simulink model "Optimal_Simulation_ICE"  (R2020a)
settings: Solver=ode45  StartTime=0.0  StopTime=6948  RelTol=1e-3
values from neighbouring files (symbols this model uses):
  diff_gear = x(7)    [Opti_sub_ICE.m]
  do_21 = x(13)    [Opti_sub_ICE.m]
  do_32 = x(14)    [Opti_sub_ICE.m]
  do_43 = x(15)    [Opti_sub_ICE.m]
  do_54 = x(16)    [Opti_sub_ICE.m]
  do_65 = x(17)    [Opti_sub_ICE.m]
  EM_gear_ratio = 4.51    [init_Opti_ICE.m]
  fifth_gear = x(5)    [Opti_sub_ICE.m]
  first_gear = x(1)    [Opti_sub_ICE.m]
  fourth_gear = x(4)    [Opti_sub_ICE.m]
  gear_eff = 0.95    [init_Opti_ICE.m]
  gear_idling_loss = 300    [init_Opti_ICE.m]
  max_CE_power = 60    [init_Opti_ICE.m]
  max_EM_power = 90    [init_Opti_ICE.m]
  max_SOC = 0.60    (= 0.6)    [init_Opti_ICE.m]
  min_SOC = 0.35    [init_Opti_ICE.m]
  second_gear = x(2)    [Opti_sub_ICE.m]
  sixth_gear = x(6)    [Opti_sub_ICE.m]
  T_CE_max = p_me_max*V_d/(2*pi*2)    [init_Opti_ICE.m]
  T_EM_max = T_EM_max * max_EM_power*1000/max_EM_power_old    [init_Opti_ICE.m]
  third_gear = x(3)    [Opti_sub_ICE.m]
  up_12 = x(8)    [Opti_sub_ICE.m]
  up_23 = x(9)    [Opti_sub_ICE.m]
  up_34 = x(10)    [Opti_sub_ICE.m]
  up_45 = x(11)    [Opti_sub_ICE.m]
  up_56 = x(12)    [Opti_sub_ICE.m]
  V_wheel_dia = 0.739    [init_Opti_ICE.m]
undefined symbols (not defined in the file or in its folder): automatic_gearbox, eta_EM_map, h, H_u, k_cs, P_aux, P_CE_cutoff, P_CE_idle, r, rho_f, T_CE_cutoff, theta_CE, theta_EM, V_CE_map, w_CE_idle, w_CE_max, w_CE_upper, w_EM_row, w_EM_upper
libraries: qss_tb_library x5
settings Model: Creator=davidci  LastModifiedBy=Rahul Pai
settings DataIOCC: LimitDataPoints=on  SaveFormat=Array  ReturnWorkspaceOutputs=off
settings OptimizationCC: BlockReduction=off  BooleanDataType=off  LifeSpan=inf
settings DebuggingCC: SaveWithParameterizedLinksMsg=none  UnderspecifiedInitializationDetection=Classic  MergeDetectMultiDrivingBlocksExec=none  SignalResolutionControl=TryResolveAllWithWarning  SFUnexpectedBacktrackingDiag=warning  SFNoUnconditionalDefaultTransitionDiag=warning  SFExecutionAtInitializationDiag=none  ArithmeticOperatorsInVariantConditions=warning
settings HardwareCC: ProdBitPerPointer=32  ProdBitPerSizeT=32  ProdBitPerPtrDiffT=32  ProdLargestAtomicFloat=None  ProdIntDivRoundTo=Undefined  ProdEndianess=Unspecified  ProdWordSize=32  ProdHWDeviceType=32-bit Generic  TargetUnknown=on
settings ModelReferenceCC: PropagateSignalLabelsOutOfModel=off
settings SFSimCC: SimUseLocalCustomCode=off  CustomCodeUndefinedFunction=UseInterfaceOnly
settings RTWCC: RTWUseLocalCustomCode=off
settings CodeAppCC: StateflowObjectComments=on
settings GRTTargetCC: TargetLangStandard=C89/C90 (ANSI)
settings ConfigComp: CovMetricSettings=dw  CovHtmlReporting=on  CovSaveCumulativeToWorkspaceVar=on  CovSaveSingleToWorkspaceVar=on  CovExternalEMLEnable=off  CovSFcnEnable=off

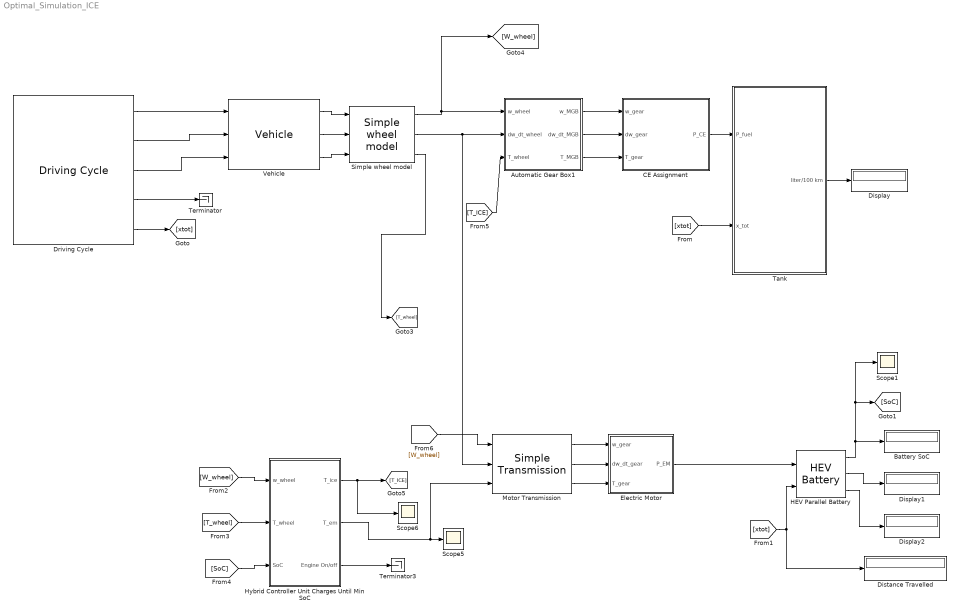
== system Optimal_Simulation_ICE ==
  Automatic Gear Box1 : Subsystem  Tag=transmission  AncestorBlock=qss_tb_library/Gear System/Automatic Gear Box  mask(Automatic Gear Box){nog=6, i=[first_gear second_gear third_gear fourth_gear fifth_gear sixth_gear], i_diff=diff_gear, gearon=[up_12 up_23 up_34 up_45 up_56], gearoff=[do_21 do_32 do_43 do_54 do_65], d=V_wheel_dia, e_GT=gear_eff, P_GT0=gear_idling_loss, w_wheel_min=1}
      mask prompts: nog "Number of gears"; i "Gear ratio vector"; i_diff "Differential gear [-]"; gearon "Switching points for upshift [km/h]"; gearoff "Switching points for downshift [km/h]"; d "Wheel diameter"; e_GT "Efficiency [-]"; P_GT0 "Idling losses (friction) [W]"; w_wheel_min "Minimum wheel speed beyond which losses are generated [rad/s]"
      mask help:
      | This block simulates a automatic gear box, can handle up to 16 gears.
      |
      | Input:
      | =====
      | 	w_wheel	Speed of the wheel [rad/s]
      | 	dw_dt_wheel	Acceleration of the wheel [rad/s^2],
      | 	T_wheel	Torque on the wheel [Nm]
      | 	i	Gear number [-]
      |
      | Output:
      | ======
      | 	w_MGB	Speed of the fly wheel [rad/s]
      | 	dw_dt_MGB	Acceleration of the fly wheel [rad/s^2]
      | 	T_MGB	Torque on the fly wheel [Nm]
      |
      | Number of gears:
      | ======
      | Specify the number of forward gears
      |
      | Shifting points for upshift:
      | ======
      | Vector specifying the velocity for shifting
      | [first_to_second_gear    second_to_third_gear    ....]
      | The number of elements in the vector should be Number of gears - 1.
      |
      | Shifting points for udownshift:
      | ======
      | Simular to upshift
      | [second_to_first_gear    third_to_second_gear    ....]
      mask init:
      | init_AGB;
  Battery SoC : Display
  CE Assignment : Subsystem  Tag=combustion engine  AncestorBlock=qss_tb_library/Energy Converter/CE Assignment  mask(Combustion Engine (based on consumption map)){engine_type=Gasoline, P_ice=max_CE_power, ENABLE_FUEL_CUTOFF=off}
      mask prompts: engine_type "Engine type"; P_ice "Power [kW]"; ENABLE_FUEL_CUTOFF "Enable fuel cutoff"
      mask help:
      | This block simulates the behaviour of a combustion engine. The block is based on consumption maps for medium sized passenger cars.
      |
      | NA Gasoline:
      | max power @ 5000 rpm
      | max torque @ 3000 rpm
      |
      | Small Diesel:
      | max power @ 4500 rpm
      | max torque @ 2000 rpm
      |
      | Large Diesel:
      | max power @ 1500 rpm
      | max torque @ 1500 rpm
      |
      |
      | Input:
      | =====
      | 	w_gear		Speed of the fly wheel [rad/s]
      | 	dw_gear	Acceleration of the fly wheel [rad/s^2]
      | 	T_gear		Torque on the fly wheel [Nm]
      |
      | Output:
      | ======
      | 	P_CE		Power produced by the combustion engine [W]
      mask init:
      | init_AssCE_map;
      mask TypeOptions engine_type: Gasoline | Small Diesel | Large Diesel
  Display : Display
  Display1 : Display
  Display2 : Display
  Distance Travelled : Display
      settings: Format=decimal (Stored Integer)
  Driving Cycle : qss_tb_library/Driving Cycle/Driving Cycle  Tag=cycle  cyclename1=Assignment_2_cycle  stepsize=1  autostop=on
  Electric Motor : Subsystem  AncestorBlock=qss_tb_library/Energy Converter/EM Assignment  mask(Electric Motor){P_em=max_EM_power}
      mask prompts: P_em "Power [kW]"
      mask help:
      | This block simulates the behaviour of an electric motor. The block is based on an efficiency map. The map is located in the Data/EnergyConvertter/ElectricMotor directory.
      |
      | Maximum speed och the electric motor is 6000 rpm
      | Field weakening region starts at 1500 rpm
      | Maximum mechanical power is at 2150 rpm
      | The maximum torque is 5.98 Nm/kW multiplied with the power you select.
      |
      | Input:
      | =====
      | 	w_gear	Speed of the motor [rad/s]
      | 	dw_dt_gear	Acceleration of the motor [rad/s^2]
      | 	T_gear	Torque of the motor [Nm]
      |
      | Output:
      | ======
      | 	P_EM	Electric Power consumed by the  motor [W]
      mask init:
      | init_EM_ass;
  HEV Parallel Battery : qss_tb_library/Energy Buffer/HEV Battery  Tag=battery  cell_series=N_series  cell_parallel=N_parallel  Q_BT_IC_rel=Init_SoC
  Hybrid Controller Unit Charges Until Min SoC : Subsystem  AncestorBlock=|  mask(Hybrid Controller Unit){}
      | qss_tb_library/Controller/Hybrid Controller Unit 
      | (Parallel, empty)
      mask help: Design your control strategy in this block.
      mask init:
      | init_HCU_parallel;
  Motor Transmission : qss_tb_library/Gear System/Simple Transmission  Tag=simple transmission  gear_ratio=EM_gear_ratio  e_GT=EM_gear_eta  P_GT0=EM_idling_loss  w_wheel_min=1
  Scope1 : Scope
  Scope5 : Scope
  Scope6 : Scope
  Simple wheel model : qss_tb_library/Vehicle/Simple wheel model  Tag=simple transmission  d_wheel=V_wheel_dia
  Tank : Subsystem  Tag=tank  AncestorBlock=qss_tb_library/Energy Source/Tank  mask(Tank){fuel=Gasoline, flag_cold_start=on}
      mask prompts: flag_cold_start "Include cold start losses"
      mask help:
      | This block integrates the power (the fuel mass flow) required by the combustion engine or the fuel cell and calculates the energy consumption in liter/100 km.
      |
      | Input:
      | =====
      | 	P_fuel	Power (fuel mass flow) required [W]
      | 	x_tot	Total distance [m]
      |
      | Output:
      | ======
      | 	V	Fuel consumption [liter/100 km]
      mask init:
      | init_tank;
      mask TypeOptions fuel: Gasoline | Diesel | Hydrogen
  Terminator : Terminator
  Terminator3 : Terminator
  Vehicle : qss_tb_library/Vehicle/Vehicle  Tag=vehicle  m_f=V_Mass  A_f=V_area  cw=V_d  mu=V_RRC  k_inertia=V_Rotating
  wires:
  Tank/1(liter/100 km) -> Display/1
  Driving Cycle/1 -> Vehicle/1
  Driving Cycle/2 -> Vehicle/2
  CE Assignment/1(P_CE) -> Tank/1(P_fuel)
  Driving Cycle/4 -> Terminator/1
  Driving Cycle/3 -> Vehicle/3
  Vehicle/1 -> Simple wheel model/1
  Vehicle/2 -> Simple wheel model/2
  Vehicle/3 -> Simple wheel model/3
  Automatic Gear Box1/3(T_MGB) -> CE Assignment/3(T_gear)
  Automatic Gear Box1/2(dw_dt_MGB) -> CE Assignment/2(dw_gear)
  Automatic Gear Box1/1(w_MGB) -> CE Assignment/1(w_gear)
  Simple wheel model/1 -> Automatic Gear Box1/1(w_wheel), [W_wheel]
  Simple wheel model/3 -> [T_wheel]
  Driving Cycle/5 -> [xtot]
  HEV Parallel Battery/3 -> Display2/1
  Motor Transmission/3 -> Electric Motor/3(T_gear)
  Motor Transmission/1 -> Electric Motor/1(w_gear)
  Hybrid Controller Unit Charges Until Min SoC/3(Engine On/off) -> Terminator3/1
  Motor Transmission/2 -> Electric Motor/2(dw_dt_gear)
  [xtot] -> HEV Parallel Battery/2, Distance Travelled/1
  Hybrid Controller Unit Charges Until Min SoC/2(T_em) -> Motor Transmission/3, Scope5/1
  Hybrid Controller Unit Charges Until Min SoC/1(T_ice) -> Scope6/1, [T_ICE]
  [SoC] -> Hybrid Controller Unit Charges Until Min SoC/3(SoC)
  Simple wheel model/2 -> Automatic Gear Box1/2(dw_dt_wheel), Motor Transmission/2
  HEV Parallel Battery/1 -> Scope1/1, [SoC], Battery SoC/1
  Electric Motor/1(P_EM) -> HEV Parallel Battery/1
  [W_wheel] -> Hybrid Controller Unit Charges Until Min SoC/1(w_wheel)
  [W_wheel] -> Motor Transmission/1
  [T_wheel] -> Hybrid Controller Unit Charges Until Min SoC/2(T_wheel)
  HEV Parallel Battery/2 -> Display1/1
  [T_ICE] -> Automatic Gear Box1/3(T_wheel)
  [xtot] -> Tank/2(x_tot)

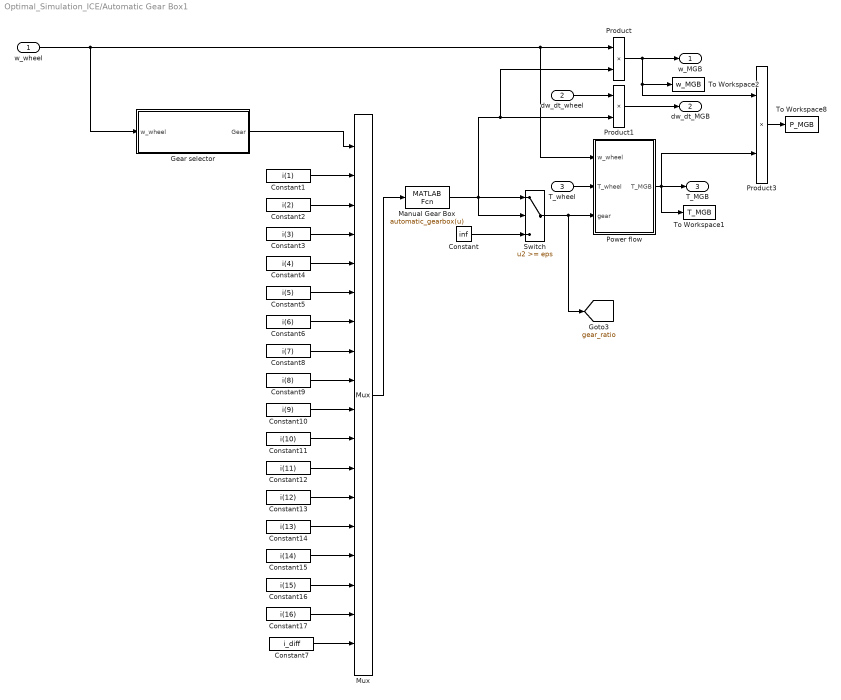
== system Optimal_Simulation_ICE/Automatic Gear Box1 ==
  w_wheel : Inport
  dw_dt_wheel : Inport  Port=2
  T_wheel : Inport  Port=3
  Constant : Constant  Value=inf
  Constant1 : Constant  Value=i(1)
  Constant10 : Constant  Value=i(9)
  Constant11 : Constant  Value=i(10)
  Constant12 : Constant  Value=i(11)
  Constant13 : Constant  Value=i(12)
  Constant14 : Constant  Value=i(13)
  Constant15 : Constant  Value=i(14)
  Constant16 : Constant  Value=i(15)
  Constant17 : Constant  Value=i(16)
  Constant2 : Constant  Value=i(2)
  Constant3 : Constant  Value=i(3)
  Constant4 : Constant  Value=i(4)
  Constant5 : Constant  Value=i(5)
  Constant6 : Constant  Value=i(6)
  Constant7 : Constant  Value=i_diff
  Constant8 : Constant  Value=i(7)
  Constant9 : Constant  Value=i(8)
  Gear selector : Subsystem
  Manual Gear Box : MATLABFcn  MATLABFcn=automatic_gearbox(u)  OutputDimensions=1
  Mux : Mux  Inputs=18
  Power flow : Subsystem
  Product : Product  InputSameDT=on  RndMeth=Zero  SaturateOnIntegerOverflow=on  OutDataTypeStr=Inherit: Same as first input
  Product1 : Product  InputSameDT=on  RndMeth=Zero  SaturateOnIntegerOverflow=on  OutDataTypeStr=Inherit: Same as first input
  Product3 : Product  InputSameDT=on  RndMeth=Zero  SaturateOnIntegerOverflow=on  OutDataTypeStr=Inherit: Same as first input
  Switch : Switch  Threshold=eps  SaturateOnIntegerOverflow=on  InputSameDT=on
  To Workspace1 : ToWorkspace  VariableName=T_MGB  SampleTime=-1
  To Workspace2 : ToWorkspace  VariableName=w_MGB  SampleTime=-1
  To Workspace8 : ToWorkspace  VariableName=P_MGB  SampleTime=-1
  w_MGB : Outport  InitialOutput=0
  dw_dt_MGB : Outport  Port=2  InitialOutput=0
  T_MGB : Outport  Port=3  InitialOutput=0
  tag scope: gear_ratio=global
  wires:
  Constant17/1 -> Mux/17
  Constant16/1 -> Mux/16
  Constant15/1 -> Mux/15
  Constant14/1 -> Mux/14
  Constant13/1 -> Mux/13
  Constant12/1 -> Mux/12
  Constant11/1 -> Mux/11
  Constant10/1 -> Mux/10
  Constant9/1 -> Mux/9
  Constant8/1 -> Mux/8
  Constant7/1 -> Mux/18
  Power flow/1(T_MGB) -> T_MGB/1, Product3/2, To Workspace1/1
  Product/1 -> w_MGB/1, Product3/1, To Workspace2/1
  Constant/1 -> Switch/3
  w_wheel/1 -> Gear selector/1(w_wheel), Product/1, Power flow/1(w_wheel)
  Product1/1 -> dw_dt_MGB/1
  dw_dt_wheel/1 -> Product1/1
  Manual Gear Box/1 -> Product/2, Product1/2, Switch/2, Switch/1
  Product3/1 -> To Workspace8/1
  Switch/1 -> [gear_ratio], Power flow/3(gear)
  T_wheel/1 -> Power flow/2(T_wheel)
  Constant1/1 -> Mux/2
  Constant2/1 -> Mux/3
  Constant3/1 -> Mux/4
  Constant4/1 -> Mux/5
  Constant5/1 -> Mux/6
  Constant6/1 -> Mux/7
  Gear selector/1(Gear) -> Mux/1
  Mux/1 -> Manual Gear Box/1

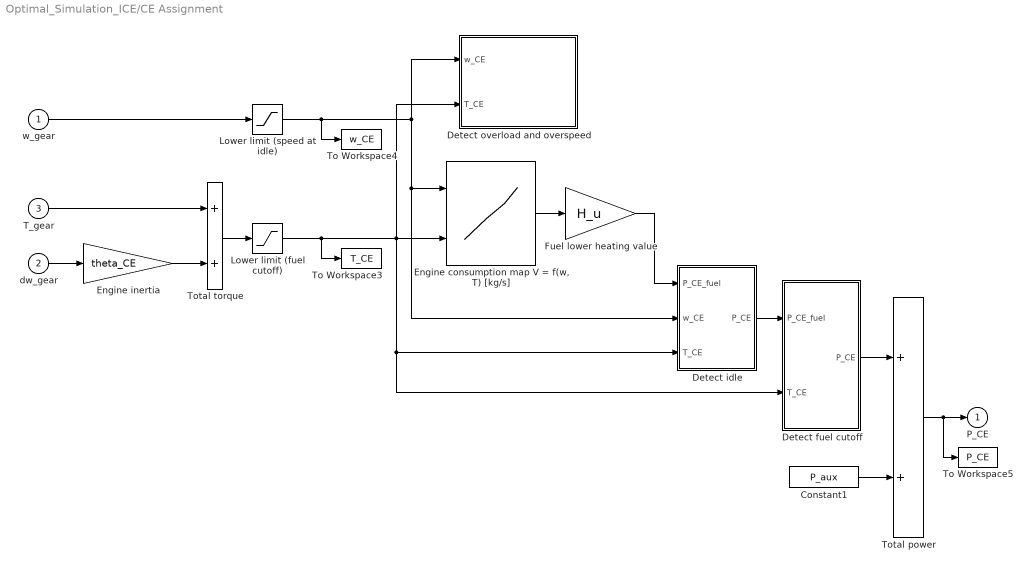
== system Optimal_Simulation_ICE/CE Assignment ==
  w_gear : Inport
  dw_gear : Inport  Port=2
  T_gear : Inport  Port=3
  Constant1 : Constant  Value=P_aux
  Detect fuel cutoff : Subsystem
  Detect idle : Subsystem
  Detect overload and overspeed : Subsystem
  "Engine consumption map V = f(w, T) [kg/s]" : Lookup2D  RowIndex=w_CE_row  ColumnIndex=T_CE_col  Table=V_CE_map
  Engine inertia : Gain  Gain=theta_CE  SaturateOnIntegerOverflow=on  OutDataTypeStr=Inherit: Same as input  ParamDataTypeStr=Inherit: Same as input
  Fuel lower heating value : Gain  Gain=H_u  SaturateOnIntegerOverflow=on  OutDataTypeStr=Inherit: Same as input  ParamDataTypeStr=Inherit: Same as input
  Lower limit (fuel cutoff) : Saturate  UpperLimit=inf  LowerLimit=T_CE_cutoff
  Lower limit (speed at idle) : Saturate  UpperLimit=inf  LowerLimit=w_CE_idle
  To Workspace3 : ToWorkspace  VariableName=T_CE  SampleTime=-1
  To Workspace4 : ToWorkspace  VariableName=w_CE  SampleTime=-1
  To Workspace5 : ToWorkspace  VariableName=P_CE  SampleTime=-1
  Total power : Sum  InputSameDT=on  SaturateOnIntegerOverflow=on  OutDataTypeStr=Inherit: Same as first input
  Total torque : Sum  InputSameDT=on  SaturateOnIntegerOverflow=on  OutDataTypeStr=Inherit: Same as first input
  P_CE : Outport  InitialOutput=0
  wires:
  T_gear/1 -> Total torque/1
  dw_gear/1 -> Engine inertia/1
  Total torque/1 -> Lower limit (fuel cutoff)/1
  Engine inertia/1 -> Total torque/2
  Lower limit (speed at idle)/1 -> Detect overload and overspeed/1(w_CE), Detect idle/2(w_CE), "Engine consumption map V = f(w, T) [kg/s]"/1, To Workspace4/1
  w_gear/1 -> Lower limit (speed at idle)/1
  Fuel lower heating value/1 -> Detect idle/1(P_CE_fuel)
  Detect idle/1(P_CE) -> Detect fuel cutoff/1(P_CE_fuel)
  "Engine consumption map V = f(w, T) [kg/s]"/1 -> Fuel lower heating value/1
  Detect fuel cutoff/1(P_CE) -> Total power/1
  Total power/1 -> P_CE/1, To Workspace5/1
  Constant1/1 -> Total power/2
  Lower limit (fuel cutoff)/1 -> Detect overload and overspeed/2(T_CE), "Engine consumption map V = f(w, T) [kg/s]"/2, Detect idle/3(T_CE), Detect fuel cutoff/2(T_CE), To Workspace3/1

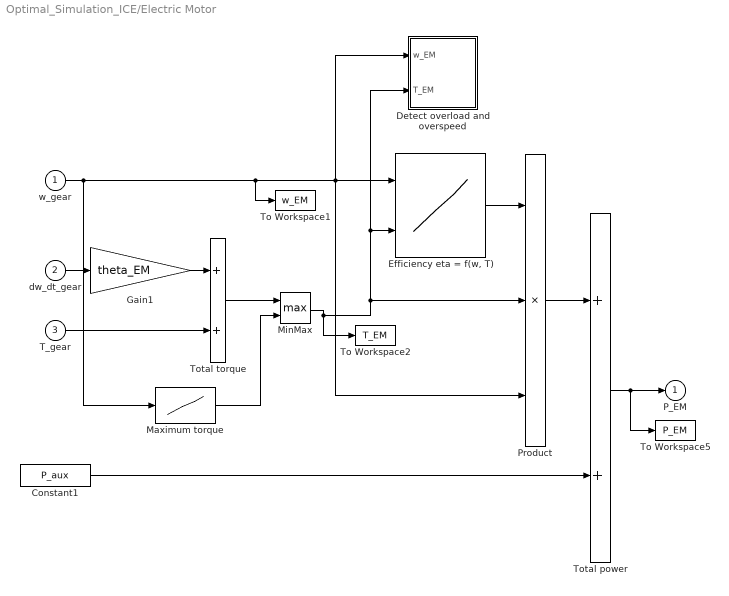
== system Optimal_Simulation_ICE/Electric Motor ==
  w_gear : Inport
  dw_dt_gear : Inport  Port=2
  T_gear : Inport  Port=3
  Constant1 : Constant  Value=P_aux
  Detect overload and overspeed : Subsystem
  "Efficiency eta = f(w, T)" : Lookup2D  RowIndex=w_EM_row  ColumnIndex=T_EM_col  Table=eta_EM_map
  Gain1 : Gain  Gain=theta_EM  SaturateOnIntegerOverflow=on  OutDataTypeStr=Inherit: Same as input  ParamDataTypeStr=Inherit: Same as input
  Maximum torque : Lookup  InputValues=w_EM_row  Table=-T_EM_max  SaturateOnIntegerOverflow=on
  MinMax : MinMax  Function=max  Inputs=2
  Product : Product  Inputs=3  InputSameDT=on  RndMeth=Zero  SaturateOnIntegerOverflow=on  OutDataTypeStr=Inherit: Same as first input
  To Workspace1 : ToWorkspace  VariableName=w_EM  SampleTime=-1
  To Workspace2 : ToWorkspace  VariableName=T_EM  SampleTime=-1
  To Workspace5 : ToWorkspace  VariableName=P_EM  SampleTime=-1
  Total power : Sum  InputSameDT=on  SaturateOnIntegerOverflow=on  OutDataTypeStr=Inherit: Same as first input
  Total torque : Sum  InputSameDT=on  SaturateOnIntegerOverflow=on  OutDataTypeStr=Inherit: Same as first input
  P_EM : Outport  InitialOutput=0
  wires:
  Total power/1 -> To Workspace5/1, P_EM/1
  Product/1 -> Total power/1
  Constant1/1 -> Total power/2
  MinMax/1 -> To Workspace2/1, Product/2, "Efficiency eta = f(w, T)"/2, Detect overload and overspeed/2(T_EM)
  Gain1/1 -> Total torque/1
  T_gear/1 -> Total torque/2
  dw_dt_gear/1 -> Gain1/1
  "Efficiency eta = f(w, T)"/1 -> Product/1
  w_gear/1 -> Maximum torque/1, To Workspace1/1, Product/3, "Efficiency eta = f(w, T)"/1, Detect overload and overspeed/1(w_EM)
  Maximum torque/1 -> MinMax/2
  Total torque/1 -> MinMax/1

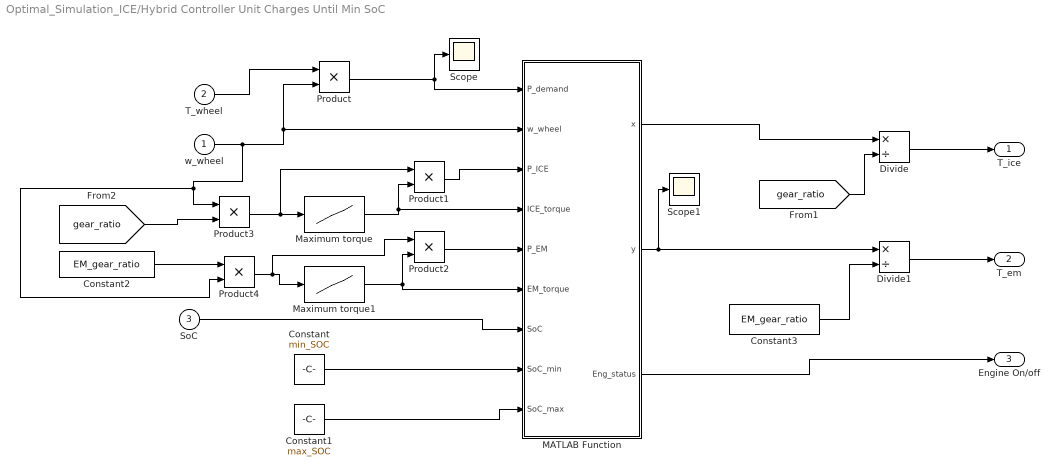
== system Optimal_Simulation_ICE/Hybrid Controller Unit Charges Until Min SoC ==
  w_wheel : Inport
  T_wheel : Inport  Port=2
  SoC : Inport  Port=3
  Constant : Constant  Value=min_SOC
  Constant1 : Constant  Value=max_SOC
  Constant2 : Constant  Value=EM_gear_ratio
  Constant3 : Constant  Value=EM_gear_ratio
  Divide : Product  Inputs=*/
  Divide1 : Product  Inputs=*/
  MATLAB Function : MATLAB Function  TreatAsAtomicUnit=on
  Maximum torque : Lookup  InputValues=w_CE_max  Table=T_CE_max  SaturateOnIntegerOverflow=on
  Maximum torque1 : Lookup  InputValues=w_EM_row  Table=T_EM_max  SaturateOnIntegerOverflow=on
  Product{,1..4} (5 alike) : Product
  Scope : Scope
  Scope1 : Scope
  T_ice : Outport  InitialOutput=0
  T_em : Outport  Port=2  InitialOutput=0
  Engine On/off : Outport  Port=3  InitialOutput=0
  wires:
  MATLAB Function/1(x) -> Divide/1
  MATLAB Function/2(y) -> Scope1/1, Divide1/1
  MATLAB Function/3(Eng_status) -> Engine On/off/1
  T_wheel/1 -> Product/1
  Product/1 -> Scope/1, MATLAB Function/1(P_demand)
  Maximum torque/1 -> Product1/2, MATLAB Function/4(ICE_torque)
  Product1/1 -> MATLAB Function/3(P_ICE)
  Maximum torque1/1 -> Product2/2, MATLAB Function/6(EM_torque)
  Product2/1 -> MATLAB Function/5(P_EM)
  SoC/1 -> MATLAB Function/7(SoC)
  Constant/1 -> MATLAB Function/8(SoC_min)
  Constant1/1 -> MATLAB Function/9(SoC_max)
  Product3/1 -> Product1/1, Maximum torque/1
  [gear_ratio] -> Product3/2
  [gear_ratio] -> Divide/2
  Constant2/1 -> Product4/1
  w_wheel/1 -> Product3/1, Product4/2, Product/2, MATLAB Function/2(w_wheel)
  Product4/1 -> Product2/1, Maximum torque1/1
  Constant3/1 -> Divide1/2
  Divide1/1 -> T_em/1
  Divide/1 -> T_ice/1

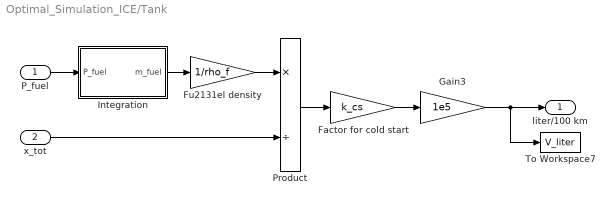
== system Optimal_Simulation_ICE/Tank ==
  P_fuel : Inport
  x_tot : Inport  Port=2
  Factor for cold start : Gain  Gain=k_cs  SaturateOnIntegerOverflow=on  OutDataTypeStr=Inherit: Same as input  ParamDataTypeStr=Inherit: Same as input
  Fu2131el density : Gain  Gain=1/rho_f  SaturateOnIntegerOverflow=on  OutDataTypeStr=Inherit: Same as input  ParamDataTypeStr=Inherit: Same as input
  Gain3 : Gain  Gain=1e5  SaturateOnIntegerOverflow=on  OutDataTypeStr=Inherit: Same as input  ParamDataTypeStr=Inherit: Same as input
  Integration : Subsystem
  Product : Product  Inputs=*/  InputSameDT=on  RndMeth=Zero  SaturateOnIntegerOverflow=on  OutDataTypeStr=Inherit: Same as first input
  To Workspace7 : ToWorkspace  VariableName=V_liter  SampleTime=-1
  liter/100 km : Outport  InitialOutput=0
  wires:
  Factor for cold start/1 -> Gain3/1
  Product/1 -> Factor for cold start/1
  Fu2131el density/1 -> Product/1
  Gain3/1 -> To Workspace7/1, liter/100 km/1
  Integration/1(m_fuel) -> Fu2131el density/1
  x_tot/1 -> Product/2
  P_fuel/1 -> Integration/1(P_fuel)

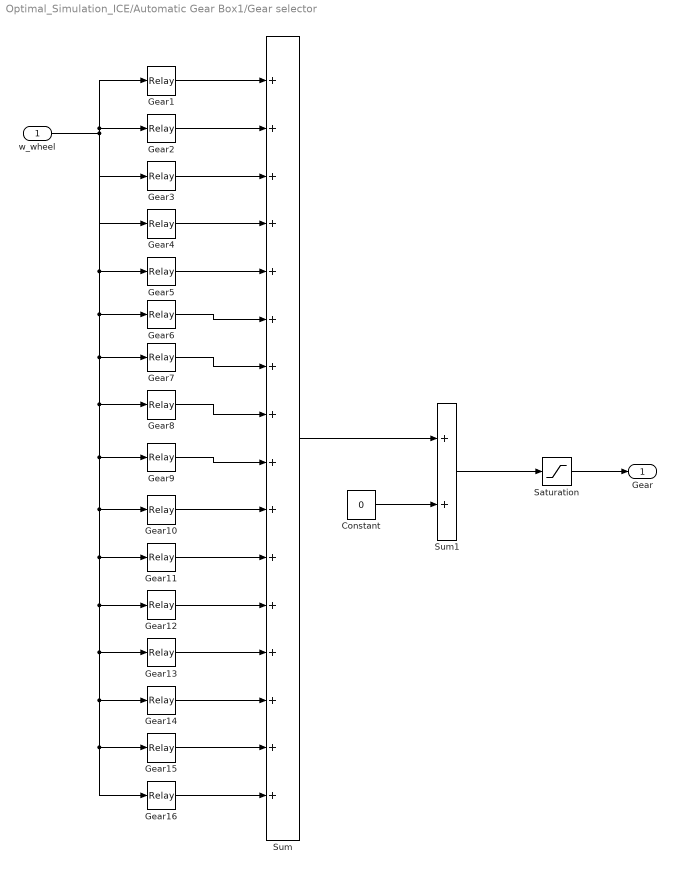
== system Optimal_Simulation_ICE/Automatic Gear Box1/Gear selector ==
  w_wheel : Inport
  Constant : Constant  Value=0
  Gear1 : Relay  OffSwitchValue=0
  Gear10 : Relay  OnSwitchValue=gearon(9)/3.6/r  OffSwitchValue=gearoff(9)/3.6/r
  Gear11 : Relay  OnSwitchValue=gearon(10)/3.6/r  OffSwitchValue=gearoff(10)/3.6/r
  Gear12 : Relay  OnSwitchValue=gearon(11)/3.6/r  OffSwitchValue=gearoff(11)/3.6/r
  Gear13 : Relay  OnSwitchValue=gearon(12)/3.6/r  OffSwitchValue=gearoff(12)/3.6/r
  Gear14 : Relay  OnSwitchValue=gearon(13)/3.6/r  OffSwitchValue=gearoff(13)/3.6/r
  Gear15 : Relay  OnSwitchValue=gearon(14)/3.6/r  OffSwitchValue=gearoff(14)/3.6/r
  Gear16 : Relay  OnSwitchValue=gearon(15)/3.6/r  OffSwitchValue=gearoff(15)/3.6/r
  Gear2 : Relay  OnSwitchValue=gearon(1)/3.6/r  OffSwitchValue=gearoff(1)/3.6/r
  Gear3 : Relay  OnSwitchValue=gearon(2)/3.6/r  OffSwitchValue=gearoff(2)/3.6/r
  Gear4 : Relay  OnSwitchValue=gearon(3)/3.6/r  OffSwitchValue=gearoff(3)/3.6/r
  Gear5 : Relay  OnSwitchValue=gearon(4)/3.6/r  OffSwitchValue=gearoff(4)/3.6/r
  Gear6 : Relay  OnSwitchValue=gearon(5)/3.6/r  OffSwitchValue=gearoff(5)/3.6/r
  Gear7 : Relay  OnSwitchValue=gearon(6)/3.6/r  OffSwitchValue=gearoff(6)/3.6/r
  Gear8 : Relay  OnSwitchValue=gearon(7)/3.6/r  OffSwitchValue=gearoff(7)/3.6/r
  Gear9 : Relay  OnSwitchValue=gearon(8)/3.6/r  OffSwitchValue=gearoff(8)/3.6/r
  Saturation : Saturate  UpperLimit=nog  LowerLimit=0
  Sum : Sum  Inputs=16  SaturateOnIntegerOverflow=on
  Sum1 : Sum  Inputs=2  SaturateOnIntegerOverflow=on
  Gear : Outport
  wires:
  Saturation/1 -> Gear/1
  Gear6/1 -> Sum/6
  Gear7/1 -> Sum/7
  Gear8/1 -> Sum/8
  Gear9/1 -> Sum/9
  Gear10/1 -> Sum/10
  Gear11/1 -> Sum/11
  Gear12/1 -> Sum/12
  Gear13/1 -> Sum/13
  Gear14/1 -> Sum/14
  Gear15/1 -> Sum/15
  Gear16/1 -> Sum/16
  Gear5/1 -> Sum/5
  w_wheel/1 -> Gear16/1, Gear15/1, Gear14/1, Gear13/1, Gear12/1, Gear11/1, Gear10/1, Gear9/1, Gear8/1, Gear7/1, Gear6/1, Gear5/1, Gear1/1, Gear2/1, Gear3/1, Gear4/1
  Gear1/1 -> Sum/1
  Gear2/1 -> Sum/2
  Gear3/1 -> Sum/3
  Gear4/1 -> Sum/4
  Sum/1 -> Sum1/1
  Sum1/1 -> Saturation/1
  Constant/1 -> Sum1/2

== system Optimal_Simulation_ICE/Automatic Gear Box1/Power flow ==
  w_wheel : Inport
  T_wheel : Inport  Port=2
  gear : Inport  Port=3
  "Engine -> Wheel" : Subsystem
  Switch1 : Switch  SaturateOnIntegerOverflow=on  InputSameDT=on
  "Wheel -> Engine" : Subsystem
  T_MGB : Outport  InitialOutput=0
  wires:
  w_wheel/1 -> "Wheel -> Engine"/1(w_wheel), "Engine -> Wheel"/1(w_wheel)
  gear/1 -> "Wheel -> Engine"/3(gear), "Engine -> Wheel"/3(gear)
  "Wheel -> Engine"/1(T_MGB-) -> Switch1/3
  T_wheel/1 -> "Wheel -> Engine"/2(T_wheel), "Engine -> Wheel"/2(T_wheel), Switch1/2
  "Engine -> Wheel"/1(T_MGB+) -> Switch1/1
  Switch1/1 -> T_MGB/1

== system Optimal_Simulation_ICE/CE Assignment/Detect fuel cutoff ==
  P_CE_fuel : Inport
  T_CE : Inport  Port=2
  Constant1 : Constant  Value=ENABLE_FUEL_CUTOFF
  Constant3 : Constant  Value=P_CE_cutoff
  Decision : Switch  Threshold=0.5
  Detect fuel cutoff : Switch  Threshold=T_CE_cutoff + 0.01  SaturateOnIntegerOverflow=on  InputSameDT=on
  P_CE : Outport
  wires:
  Constant3/1 -> Detect fuel cutoff/3
  T_CE/1 -> Detect fuel cutoff/2
  P_CE_fuel/1 -> Detect fuel cutoff/1, Decision/3
  Detect fuel cutoff/1 -> Decision/1
  Constant1/1 -> Decision/2
  Decision/1 -> P_CE/1

== system Optimal_Simulation_ICE/CE Assignment/Detect idle ==
  P_CE_fuel : Inport
  w_CE : Inport  Port=2
  T_CE : Inport  Port=3
  Constant3 : Constant  Value=P_CE_idle
  Idle detection : Fcn  Expr=(u(1) <= w_CE_idle) * (u(2) <= T_CE_idle)
  Mux : Mux  Inputs=2
  Switch2 : Switch  Threshold=0.5  SaturateOnIntegerOverflow=on  InputSameDT=on
  P_CE : Outport  InitialOutput=0
  wires:
  Mux/1 -> Idle detection/1
  T_CE/1 -> Mux/2
  w_CE/1 -> Mux/1
  Idle detection/1 -> Switch2/2
  P_CE_fuel/1 -> Switch2/3
  Switch2/1 -> P_CE/1
  Constant3/1 -> Switch2/1

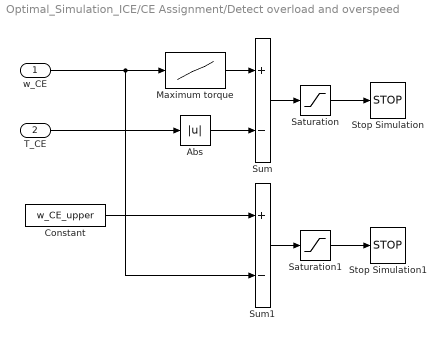
== system Optimal_Simulation_ICE/CE Assignment/Detect overload and overspeed ==
  w_CE : Inport
  T_CE : Inport  Port=2
  Abs : Abs  SaturateOnIntegerOverflow=on
  Constant : Constant  Value=w_CE_upper
  Maximum torque : Lookup  InputValues=w_CE_max  Table=T_CE_max  SaturateOnIntegerOverflow=on
  Saturation : Saturate  UpperLimit=0  LowerLimit=-inf
  Saturation1 : Saturate  UpperLimit=0  LowerLimit=-inf
  Stop Simulation : Stop
  Stop Simulation1 : Stop
  Sum : Sum  Inputs=+-  InputSameDT=on  SaturateOnIntegerOverflow=on  OutDataTypeStr=Inherit: Same as first input
  Sum1 : Sum  Inputs=+-  InputSameDT=on  SaturateOnIntegerOverflow=on  OutDataTypeStr=Inherit: Same as first input
  wires:
  Sum/1 -> Saturation/1
  w_CE/1 -> Maximum torque/1, Sum1/2
  T_CE/1 -> Abs/1
  Maximum torque/1 -> Sum/1
  Abs/1 -> Sum/2
  Saturation/1 -> Stop Simulation/1
  Constant/1 -> Sum1/1
  Sum1/1 -> Saturation1/1
  Saturation1/1 -> Stop Simulation1/1

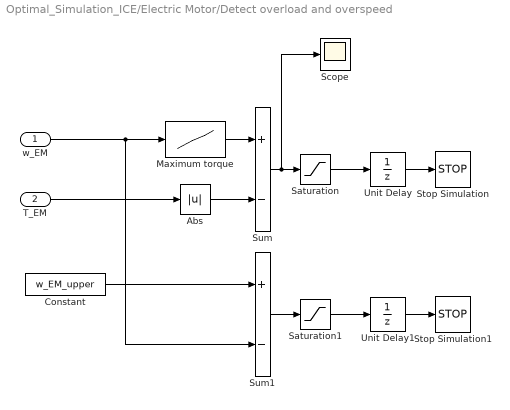
== system Optimal_Simulation_ICE/Electric Motor/Detect overload and overspeed ==
  w_EM : Inport
  T_EM : Inport  Port=2
  Abs : Abs  SaturateOnIntegerOverflow=on
  Constant : Constant  Value=w_EM_upper
  Maximum torque : Lookup  InputValues=w_EM_row  Table=T_EM_max  SaturateOnIntegerOverflow=on
  Saturation : Saturate  UpperLimit=0  LowerLimit=-inf
  Saturation1 : Saturate  UpperLimit=0  LowerLimit=-inf
  Scope : Scope
  Stop Simulation : Stop
  Stop Simulation1 : Stop
  Sum : Sum  Inputs=+-  InputSameDT=on  SaturateOnIntegerOverflow=on  OutDataTypeStr=Inherit: Same as first input
  Sum1 : Sum  Inputs=+-  InputSameDT=on  SaturateOnIntegerOverflow=on  OutDataTypeStr=Inherit: Same as first input
  Unit Delay : UnitDelay  SampleTime=-1  HasFrameUpgradeWarning=on
  Unit Delay1 : UnitDelay  SampleTime=-1  HasFrameUpgradeWarning=on
  wires:
  Sum/1 -> Scope/1, Saturation/1
  w_EM/1 -> Maximum torque/1, Sum1/2
  T_EM/1 -> Abs/1
  Maximum torque/1 -> Sum/1
  Abs/1 -> Sum/2
  Saturation/1 -> Unit Delay/1
  Constant/1 -> Sum1/1
  Sum1/1 -> Saturation1/1
  Saturation1/1 -> Unit Delay1/1
  Unit Delay/1 -> Stop Simulation/1
  Unit Delay1/1 -> Stop Simulation1/1

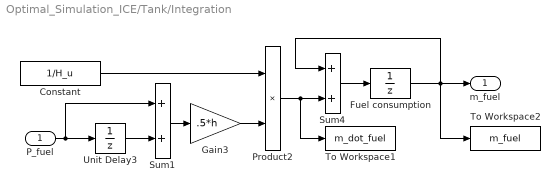
== system Optimal_Simulation_ICE/Tank/Integration ==
  P_fuel : Inport
  Constant : Constant  Value=1/H_u
  Fuel consumption : UnitDelay  SampleTime=h  HasFrameUpgradeWarning=on
  Gain3 : Gain  Gain=.5*h  SaturateOnIntegerOverflow=on  OutDataTypeStr=Inherit: Same as input  ParamDataTypeStr=Inherit: Same as input
  Product2 : Product  InputSameDT=on  RndMeth=Zero  SaturateOnIntegerOverflow=on  OutDataTypeStr=Inherit: Same as first input
  Sum1 : Sum  InputSameDT=on  SaturateOnIntegerOverflow=on  OutDataTypeStr=Inherit: Same as first input
  Sum4 : Sum  InputSameDT=on  SaturateOnIntegerOverflow=on  OutDataTypeStr=Inherit: Same as first input
  To Workspace1 : ToWorkspace  VariableName=m_dot_fuel  SampleTime=-1
  To Workspace2 : ToWorkspace  VariableName=m_fuel  SampleTime=-1
  Unit Delay3 : UnitDelay  SampleTime=h  HasFrameUpgradeWarning=on
  m_fuel : Outport  InitialOutput=0
  wires:
  Product2/1 -> To Workspace1/1, Sum4/2
  Sum4/1 -> Fuel consumption/1
  Fuel consumption/1 -> To Workspace2/1, Sum4/1, m_fuel/1
  Sum1/1 -> Gain3/1
  Unit Delay3/1 -> Sum1/2
  P_fuel/1 -> Unit Delay3/1, Sum1/1
  Gain3/1 -> Product2/2
  Constant/1 -> Product2/1

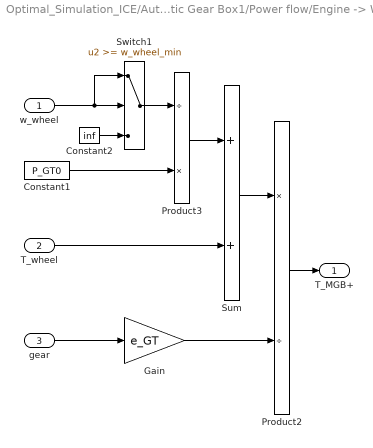
== system Optimal_Simulation_ICE/Automatic Gear Box1/Power flow/Engine -> Wheel ==
  w_wheel : Inport
  T_wheel : Inport  Port=2
  gear : Inport  Port=3
  Constant1 : Constant  Value=P_GT0
  Constant2 : Constant  Value=inf
  Gain : Gain  Gain=e_GT  SaturateOnIntegerOverflow=on  OutDataTypeStr=Inherit: Same as input  ParamDataTypeStr=Inherit: Same as input
  Product2 : Product  Inputs=*/  InputSameDT=on  RndMeth=Zero  SaturateOnIntegerOverflow=on  OutDataTypeStr=Inherit: Same as first input
  Product3 : Product  Inputs=/*  InputSameDT=on  RndMeth=Zero  SaturateOnIntegerOverflow=on  OutDataTypeStr=Inherit: Same as first input
  Sum : Sum  InputSameDT=on  SaturateOnIntegerOverflow=on  OutDataTypeStr=Inherit: Same as first input
  Switch1 : Switch  Threshold=w_wheel_min  SaturateOnIntegerOverflow=on  InputSameDT=on
  T_MGB+ : Outport  InitialOutput=0
  wires:
  T_wheel/1 -> Sum/2
  Product3/1 -> Sum/1
  Gain/1 -> Product2/2
  Product2/1 -> T_MGB+/1
  Sum/1 -> Product2/1
  w_wheel/1 -> Switch1/2, Switch1/1
  Constant2/1 -> Switch1/3
  Switch1/1 -> Product3/1
  Constant1/1 -> Product3/2
  gear/1 -> Gain/1

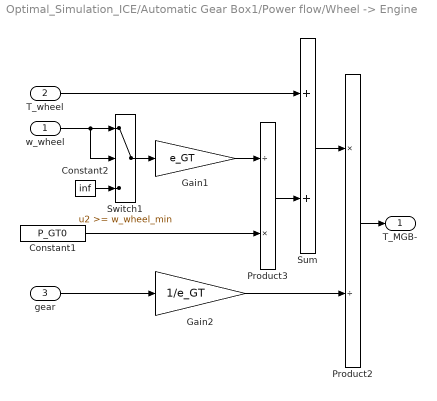
== system Optimal_Simulation_ICE/Automatic Gear Box1/Power flow/Wheel -> Engine ==
  w_wheel : Inport
  T_wheel : Inport  Port=2
  gear : Inport  Port=3
  Constant1 : Constant  Value=P_GT0
  Constant2 : Constant  Value=inf
  Gain1 : Gain  Gain=e_GT  SaturateOnIntegerOverflow=on  OutDataTypeStr=Inherit: Same as input  ParamDataTypeStr=Inherit: Same as input
  Gain2 : Gain  Gain=1/e_GT  SaturateOnIntegerOverflow=on  OutDataTypeStr=Inherit: Same as input  ParamDataTypeStr=Inherit: Same as input
  Product2 : Product  Inputs=*/  InputSameDT=on  RndMeth=Zero  SaturateOnIntegerOverflow=on  OutDataTypeStr=Inherit: Same as first input
  Product3 : Product  Inputs=/*  InputSameDT=on  RndMeth=Zero  SaturateOnIntegerOverflow=on  OutDataTypeStr=Inherit: Same as first input
  Sum : Sum  InputSameDT=on  SaturateOnIntegerOverflow=on  OutDataTypeStr=Inherit: Same as first input
  Switch1 : Switch  Threshold=w_wheel_min  SaturateOnIntegerOverflow=on  InputSameDT=on
  T_MGB- : Outport  InitialOutput=0
  wires:
  w_wheel/1 -> Switch1/1, Switch1/2
  gear/1 -> Gain2/1
  Constant2/1 -> Switch1/3
  Switch1/1 -> Gain1/1
  Constant1/1 -> Product3/2
  T_wheel/1 -> Sum/1
  Gain2/1 -> Product2/2
  Product2/1 -> T_MGB-/1
  Product3/1 -> Sum/2
  Sum/1 -> Product2/1
  Gain1/1 -> Product3/1

== matlab function Optimal_Simulation_ICE/Hybrid Controller Unit Charges Until Min SoC/MATLAB Function ==
  data: x output; y output; Eng_status output; P_demand input; w_wheel input; P_ICE input; ICE_torque input; P_EM input; EM_torque input; SoC input; SoC_min input; SoC_max input
function [x,y,Eng_status] = fcn(P_demand,w_wheel,P_ICE,ICE_torque,P_EM,EM_torque,SoC,SoC_min,SoC_max)
    if P_demand<=0
        if w_wheel==0
            y=0;
        else
            y=P_demand/w_wheel;
        end
        x=0;
        Eng_status=0;
    else
        if SoC<SoC_min
            if P_demand<P_ICE
                if P_ICE-P_demand>=P_EM
                    y=-EM_torque;
                    x=(P_demand+P_EM)/w_wheel;
                    Eng_status=1;
                else
                    x=ICE_torque;
                    y=-(P_ICE-P_demand)/w_wheel;
                    Eng_status=1;
                end
            else
               x=ICE_torque;
               y=(P_demand-P_ICE)/w_wheel;
               Eng_status=1;
            end
        elseif SoC>=SoC_min && SoC<SoC_max
            if P_demand<=P_EM
                y=P_demand/w_wheel;
                x=0;
                Eng_status=0;
            else
                y=EM_torque;
                x=(P_demand-P_EM)/w_wheel;
                Eng_status=1;
            end
        else
            if P_demand<=P_EM
                y=P_demand/w_wheel;
                x=0;
                Eng_status=0;
            else
                y=EM_torque;
                x=(P_demand-P_EM)/w_wheel;
                Eng_status=1;
            end
        end
    end
end
